simulink model "model"  (R2024b)
settings: Solver=ode15s  StartTime=0.0  StopTime=5  MaxStep=0.01  RelTol=1e-3
StartFcn:
  | try, dp_ui_lock(PENDULUM_APP_FIG,true); catch, end
StopFcn:
  | try, dp_ui_lock(PENDULUM_APP_FIG,false); catch, end; try, dp_plot(PENDULUM_APP_FIG,'stop'); catch, end
values from neighbouring files (symbols this model uses):
  g = p.g    [dp_dynamics.m]    (also in ui_update_model_info.m = safeField(p,'g',9.81))
  K = lqr(A,B,Q,R)    [dp_lqr_calc.m]
  l1 = p.l1    [dp_dynamics.m]    (also in ui_update_model_info.m = safeField(p,'l1',0.50))
  l2 = p.l2    [dp_dynamics.m]    (also in ui_update_model_info.m = safeField(p,'l2',0.50))
  M = p.M    [dp_dynamics.m]    (also in ui_update_cart_params.m = 1; ui_update_model_info.m = safeField(p,'M',1.0))
  m1 = p.m1    [dp_dynamics.m]    (also in ui_update_model_info.m = safeField(p,'m1',0.10))
  m2 = p.m2    [dp_dynamics.m]    (also in ui_update_model_info.m = safeField(p,'m2',0.10))
  mode = floor(mode + 0.5)    [dp_setup.m]
  th_off = tmp    [dp_hyst_window.m]    (also in dp_model_init.m = th_on - hyst_delta; dp_reset.m = th_on - hyst_delta)
  th_on = th_off    [dp_hyst_window.m]    (also in dp_model_init.m = cfg.hyst.th_on; dp_reset.m = cfg.hyst.th_on; ui_update_hysteresis.m = app.hyst.th_on)
libraries: vrlib x1
settings Model: Creator=Lenovo  LastModifiedBy=Lenovo
settings DataIOCC: SaveOutput=off  SignalLogging=off  DSMLogging=off  VisualizeSimOutput=off  SaveTime=off

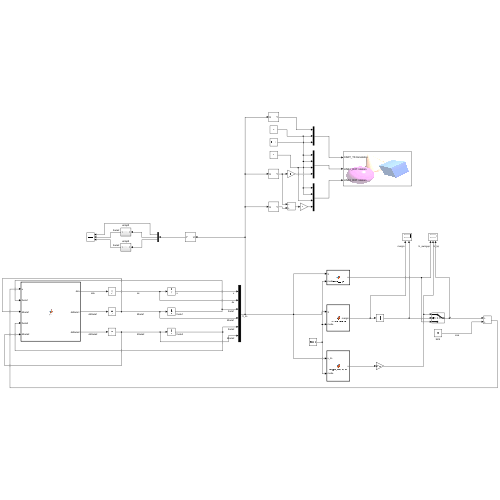
[thumbnail: Simulink's stored preview of the top-level diagram]
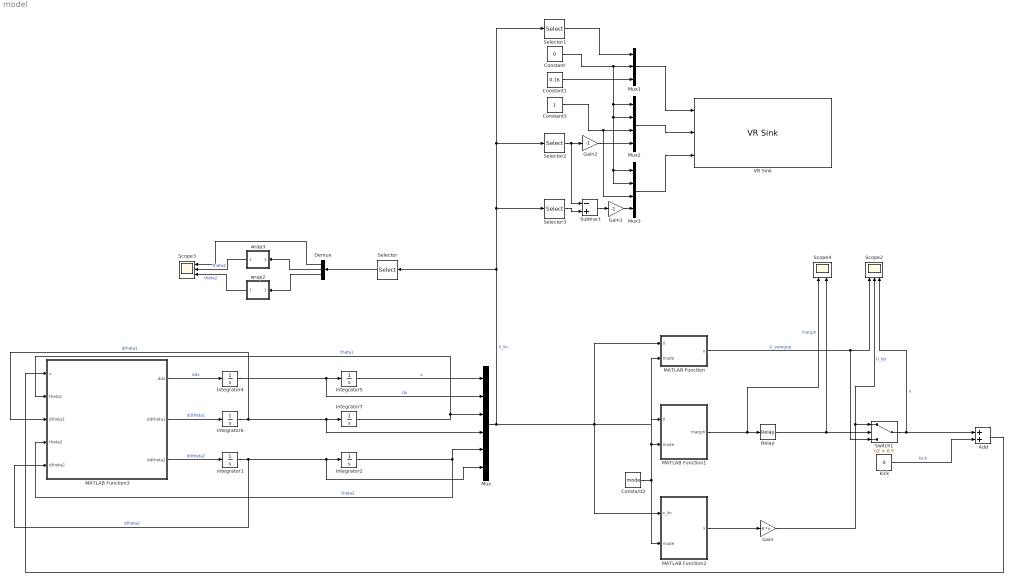
== system model ==
  Add : Sum
  Constant : Constant  Value=0
  Constant1 : Constant  Value=0.16
  Constant2 : Constant  Value=mode
  Constant3 : Constant
  Demux : Demux  Outputs=3
  Gain : Gain  Gain=-K  Multiplication=Matrix(K*u)
  Gain1 : Gain  Gain=-1
  Gain2 : Gain  Gain=-1
  Integrator{1..2,4..7} (6 alike) : Integrator
  MATLAB Function : MATLAB Function  TreatAsAtomicUnit=on
  MATLAB Function1 : MATLAB Function  TreatAsAtomicUnit=on
  MATLAB Function2 : MATLAB Function  TreatAsAtomicUnit=on
  MATLAB Function3 : MATLAB Function  TreatAsAtomicUnit=on
  Mux : Mux  Inputs=6
  Mux1 : Mux  Inputs=3
  Mux2 : Mux
  Mux3 : Mux
  Relay : Relay  OnSwitchValue=th_on  OffSwitchValue=th_off
  Scope2 : Scope  NumInputPorts=3
  Scope3 : Scope  NumInputPorts=3
  Scope4 : Scope  NumInputPorts=2
  Selector : Selector  InputPortWidth=6  IndexOptions=Index vector (dialog)  Indices=[1 3 5]  OutputSizes=1
  Selector1 : Selector  InputPortWidth=6  IndexOptions=Index vector (dialog)  Indices=[1]  OutputSizes=1
  Selector2 : Selector  InputPortWidth=6  IndexOptions=Index vector (dialog)  Indices=[3]  OutputSizes=1
  Selector3 : Selector  InputPortWidth=6  IndexOptions=Index vector (dialog)  Indices=[5]  OutputSizes=1
  Subtract : Sum  Inputs=-+
  Switch1 : Switch  Criteria=u2 > Threshold  Threshold=0.5  ZeroCross=off  SaturateOnIntegerOverflow=off  InputSameDT=off
  VR Sink : vrlib/VR Sink  InstantiateOnLoad=on  SampleTime=0.005  ViewEnable=on  RemoteChange=off  RemoteView=off  FieldsWritten=CART_TX.translation.3.1.1.double#LINK1_ROT.rotation.4.1.1.double#LINK2_ROT.rotation.4.1.1.double  WorldFileName=3DAnimation.wrl  WorldDescription=Double Inverted Pendulum - Track Only  AutoView=on  VideoDimensions=[]  AllowVariableSize=off  FigureProperties="{'Position', 'Name', 'Viewpoint', 'CameraBound', 'CameraDirection', 'CameraPosition', 'CameraUpVector', 'ZoomFactor', 'Antialiasing', 'Headlight', 'Lighting', 'Sound', 'StatusBar', 'Stereo3D', 'Stereo3DCameraOffset', 'Stereo3DHIT', 'ToolBar', 'Textures', 'Transparency', 'Triad', 'Wireframe', 'NavZones', 'NavMode', 'NavSpeed', 'CaptureFileFormat', 'CaptureFileName', 'Record2DCompressMethod', 'Record2DCompressQuality', 'Record2D', 'Record2DFileName', 'Record2DFPS', 'NavPanel'; [5.0000000000000000e+00   9.2000000000000000e+01   5.7600000000000000e+02   3.5000000000000000e+02], 'Double Inverted Pendulum - Track Only', 'Wide', 'on', [0.0000000000000000e+00   0.0000000000000000e+00  -1.0000000000000000e+00], [0.0000000000000000e+00   0.0000000000000000e+00   0.0000000000000000e+00], [0.0000000000000000e+00   1.0000000000000000e+00   0.0000000000000000e+00], [1.0000000000000000e+00], 'off', 'on', 'on', 'on', 'on', 'off', [1.0000000149011612e-01], [0.0000000000000000e+00], 'on', 'on', 'on', 'none', 'off', 'off', 'examine', 'normal', 'tif', '%f_anim_%n.tif', 'auto', [7.5000000000000000e+01], 'off', '%f_anim_%n.avi', 'auto', 'halfbar'}"
  kick : Constant  Value=0
  wrap2 : Subsystem
  wrap3 : Subsystem
  wires:
  MATLAB Function3/1(ddx) -> Integrator4/1  "ddx"
  Integrator4/1 -> Mux/2, Integrator5/1  "dx"
  Integrator6/1 -> MATLAB Function3/3(dtheta1), Mux/4, Integrator7/1  "dtheta1"
  MATLAB Function3/2(ddtheta1) -> Integrator6/1  "ddtheta1"
  Integrator1/1 -> MATLAB Function3/5(dtheta2), Mux/6, Integrator2/1  "dtheta2"
  MATLAB Function3/3(ddtheta2) -> Integrator1/1  "ddtheta2"
  Integrator7/1 -> MATLAB Function3/2(theta1), Mux/3  "theta1"
  Integrator2/1 -> Mux/5, MATLAB Function3/4(theta2)  "theta2"
  Integrator5/1 -> Mux/1  "x"
  Mux/1 -> Selector3/1, Selector1/1, Selector2/1, Selector/1, MATLAB Function/1(X), MATLAB Function1/1(X), MATLAB Function2/1(x_lin)  "X_lin"
  MATLAB Function1/1(margin) -> Scope4/1, Relay/1  "margin"
  Relay/1 -> Scope4/2, Switch1/2
  MATLAB Function/1(u) -> Switch1/3, Scope2/1  "U_swingup"
  Gain/1 -> Scope2/2, Switch1/1  "U_lqr"
  MATLAB Function2/1(x) -> Gain/1
  Switch1/1 -> Add/1, Scope2/3  "u"
  Constant2/1 -> MATLAB Function/2(mode), MATLAB Function1/2(mode), MATLAB Function2/2(mode)
  Selector/1 -> Demux/1
  Demux/1 -> Scope3/1
  Demux/2 -> wrap3/1(In1)
  Demux/3 -> wrap2/1(In1)
  wrap2/1(Output) -> Scope3/3  "theta2"
  wrap3/1(Output) -> Scope3/2  "theta2"
  Selector1/1 -> Mux1/1
  Constant/1 -> Mux2/1, Mux3/1, Mux3/2, Mux2/2, Mux1/2
  Constant1/1 -> Mux1/3
  Constant3/1 -> Mux3/3, Mux2/3
  Selector2/1 -> Subtract/1, Gain2/1
  Selector3/1 -> Subtract/2
  Mux3/1 -> VR Sink/3
  Mux2/1 -> VR Sink/2
  Mux1/1 -> VR Sink/1
  Add/1 -> MATLAB Function3/1(u)
  kick/1 -> Add/2  "kick"
  Subtract/1 -> Gain1/1
  Gain1/1 -> Mux3/4
  Gain2/1 -> Mux2/4

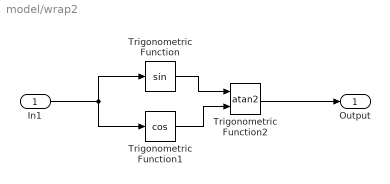
== system model/wrap2 ==
  In1 : Inport
  Trigonometric Function : Trigonometry
  Trigonometric Function1 : Trigonometry  Operator=cos
  Trigonometric Function2 : Trigonometry  Operator=atan2
  Output : Outport
  wires:
  Trigonometric Function2/1 -> Output/1
  In1/1 -> Trigonometric Function1/1, Trigonometric Function/1
  Trigonometric Function/1 -> Trigonometric Function2/1
  Trigonometric Function1/1 -> Trigonometric Function2/2

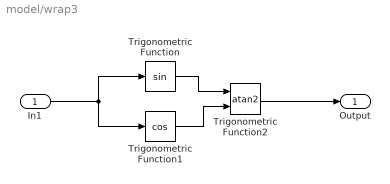
== system model/wrap3 ==
  In1 : Inport
  Trigonometric Function : Trigonometry
  Trigonometric Function1 : Trigonometry  Operator=cos
  Trigonometric Function2 : Trigonometry  Operator=atan2
  Output : Outport
  wires:
  Trigonometric Function1/1 -> Trigonometric Function2/2
  Trigonometric Function/1 -> Trigonometric Function2/1
  In1/1 -> Trigonometric Function/1, Trigonometric Function1/1
  Trigonometric Function2/1 -> Output/1

== matlab function model/MATLAB Function1 ==
  data: X input; margin output; mode input
function margin  = switch_mode(X, mode)
th1 = X(3);
th2 = X(5);

switch mode
    case 1 % (0,0)
        th1e = 0;
        th2e = 0;
    case 2 % (pi,pi)
        th1e = pi;
        th2e = pi;
    case 3 % (0,pi)
        th1e = 0;
        th2e = pi;
    case 4 % (pi,0)
        th1e = pi;
        th2e = 0;
    otherwise
        th1e = 0;
        th2e = 0;
end

e1 = atan2(sin(th1 - th1e), cos(th1 - th1e));
e2 = atan2(sin(th2 - th2e), cos(th2 - th2e));


margin = - max(abs(e1), abs(e2));   % rad
end

== matlab function model/MATLAB Function ==
  data: X input size=6; mode input; m1 parameter; m2 parameter; l2 parameter; g parameter; l1 parameter; u output
function u = swing_up(X, mode, m1, m2, l2, g, l1)

x   = X(1);  dx  = X(2);
th1 = X(3);  d1  = X(4);
th2 = X(5);  d2  = X(6);

mode = floor(mode + 0.5);

phi1 = atan2(sin(th1 - pi), cos(th1 - pi));
phi2 = atan2(sin(th2 - pi), cos(th2 - pi));

E1 = 0.5*(m1+m2)*l1^2*d1^2 + (m1+m2)*g*l1*(1 - cos(phi1));
E2 = 0.5*m2*l2^2*d2^2      +  m2*g*l2*(1 - cos(phi2));

E1_up = 2*(m1+m2)*g*l1;
E2_up = 2*(m2)*g*l2;
kE1 = 0;
kE2 = 0;

switch mode
    case 1 % (0,0) up-up
        E1_des = E1_up; E2_des = E2_up;
          kE1 = 40; kE2 = 15;
    case 2 % (pi,pi) down-down
        E1_des = 0;     E2_des = 0;
        kE1 = 17; kE2 = 13;
    case 3 % (0,pi) up-down
        E1_des = E1_up; E2_des = 0;
        kE1 = 26; kE2 = 14;
    case 4 % (pi,0) down-up
        E1_des = 0;     E2_des = E2_up;
        kE1 = 8; kE2 = 27;
    otherwise
        E1_des = E1_up; E2_des = E2_up;
end

eps = 0.4;
s1 = d1*cos(phi1);
s2 = d2*cos(phi2);

u_energy = kE1*(E1_des - E1)*tanh(s1/eps) + kE2*(E2_des - E2)*tanh(s2/eps);

kx  = 2.0;
kdx = 4.0;
u_cart = -kx*x - kdx*dx;

u = u_energy + u_cart;


end

== matlab function model/MATLAB Function2 ==
  data: x_lin input; x output; mode input
function x = angle_wrapper(x_lin, mode)

x = x_lin;

th1 = x_lin(3);
th2 = x_lin(5);

switch mode
    case 1, th1e = 0;  th2e = 0;
    case 2, th1e = pi; th2e = pi;
    case 3, th1e = 0;  th2e = pi;
    case 4, th1e = pi; th2e = 0;
    otherwise, th1e = 0; th2e = 0;
end

wrap = @(z) atan2(sin(z), cos(z));

x(3) = wrap(th1 - th1e);
x(5) = wrap(th2 - th2e);
end

== matlab function model/MATLAB Function3 ==
  data: u input; theta1 input; dtheta1 input; ddx output; ddtheta1 output; M parameter; m1 parameter; g parameter; ddtheta2 output; m2 parameter; l1 parameter; l2 parameter; theta2 input; dtheta2 input
function [ddx, ddtheta1, ddtheta2] = fcn(u, theta1, dtheta1, M, m1, g, m2, l1, l2, theta2, dtheta2) ...

s1  = sin(theta1);   c1t = cos(theta1);
s2  = sin(theta2);   c2t = cos(theta2);

d12 = theta1 - theta2;
s12 = sin(d12);
c12 = cos(d12);

Mmat = [ M + m1 + m2,        (m1 + m2)*l1*c1t,     m2*l2*c2t;
         (m1 + m2)*l1*c1t,   (m1 + m2)*l1^2,       m2*l1*l2*c12;
         m2*l2*c2t,          m2*l1*l2*c12,         m2*l2^2 ];

rhs = [ u + (m1 + m2)*l1*s1*dtheta1^2 + m2*l2*s2*dtheta2^2;
        (m1 + m2)*g*l1*s1 - m2*l1*l2*s12*dtheta2^2;
        m2*g*l2*s2 + m2*l1*l2*s12*dtheta1^2];

qdd = Mmat \ rhs;

ddx      = qdd(1);
ddtheta1 = qdd(2);
ddtheta2 = qdd(3);
end
